simulink model "Lab6_2017B5A30983P_Midpoint_Fullwave"  (R2019b)
settings: Solver=ode15s  StartTime=0.0  StopTime=0.06  RelTol=1e-3
libraries: powerlib x8, powerlib_meascontrol x2
settings Model: Creator=swaga  LastModifiedBy=swaga

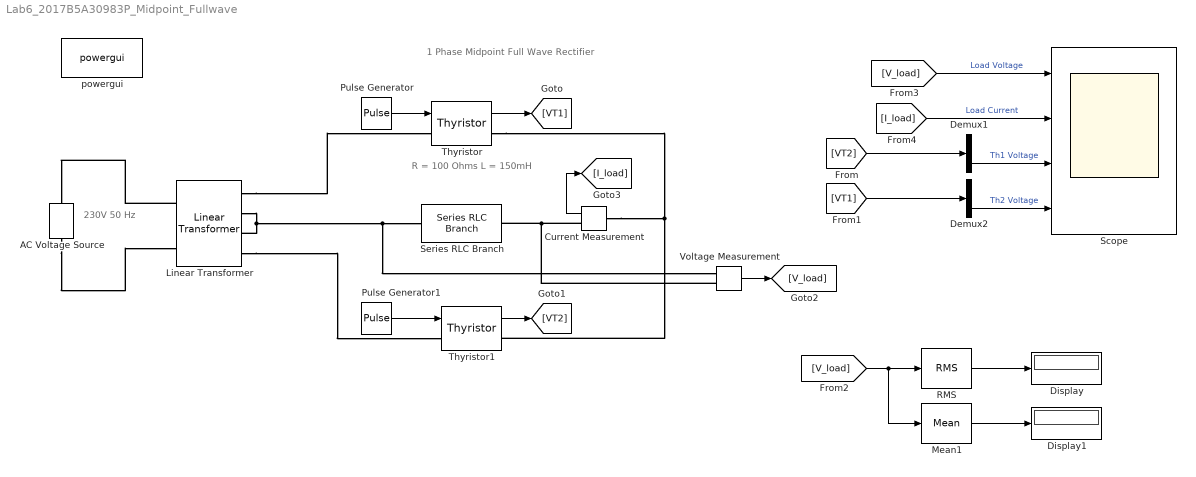
== system Lab6_2017B5A30983P_Midpoint_Fullwave ==
  note: R = 100 Ohms
      | L = 150mH
  note: 1 Phase Midpoint Full Wave Rectifier
  note: 230V
      | 50 Hz
  AC Voltage Source : powerlib/Electrical Sources/AC Voltage Source  Amplitude=230  Phase=0  Frequency=50  SampleTime=0  Measurements=None  BusType=swing  Pref=10e3  Qref=0  Qmin=-inf  Qmax=+inf
      settings: SourceProductName=Simscape Electrical
  Current Measurement : powerlib/Measurements/Current Measurement  PhasorSimulation=off  OutputType=Complex  PSBequivalent=0
      settings: SourceProductName=Simscape Electrical
  Demux1 : Demux  Outputs=2
  Demux2 : Demux  Outputs=2
  Display : Display
  Display1 : Display
  Linear Transformer : powerlib/Elements/Linear Transformer  UNITS=pu  NominalPower=[250e6 50]  winding1=[230 0.002 0.08]  winding2=[12 0.002 0]  ThreeWindings=on  winding3=[12 0.002 0]  RmLm=[ 500 500 ]  Measurements=None  DataType=off
      settings: SourceProductName=Simscape Electrical
  Mean1 : powerlib_meascontrol/Measurements/Mean  Freq=50  Vinit=0  Ts=0
      settings: SourceProductName=Simscape Electrical
  Pulse Generator : DiscretePulseGenerator  PulseType=Time based  Period=0.02  PulseWidth=5  PhaseDelay=2.5e-3
  Pulse Generator1 : DiscretePulseGenerator  PulseType=Time based  Period=0.02  PulseWidth=5  PhaseDelay=12.5e-3
  RMS : powerlib_meascontrol/Measurements/RMS  TrueRMS=on  Freq=50  RMSInit=120  Ts=0
      settings: SourceProductName=Simscape Electrical
  Scope : Scope  NumInputPorts=4
  Series RLC Branch : powerlib/Elements/Series RLC Branch  LConnTagsString=__new0  RConnTagsString=__new0  BranchType=R  Resistance=100  Inductance=150e-3  SetiL0=off  InitialCurrent=0  Capacitance=1e-6  Setx0=off  InitialVoltage=0  Measurements=None
      settings: SourceProductName=Simscape Electrical
  Thyristor : powerlib/Power Electronics/Thyristor  Ron=0.001  Lon=0  Vf=0.8  IC=0  Rs=500  Cs=250e-9  Measurements=on
      settings: SourceProductName=Simscape Electrical
  Thyristor1 : powerlib/Power Electronics/Thyristor  Ron=0.001  Lon=0  Vf=0.8  IC=0  Rs=500  Cs=250e-9  Measurements=on
      settings: SourceProductName=Simscape Electrical
  Voltage Measurement : powerlib/Measurements/Voltage Measurement  PhasorSimulation=off  OutputType=Complex  PSBequivalent=0
      settings: SourceProductName=Simscape Electrical
  powergui : powerlib/powergui  Priority=1  SimulationMode=Continuous  SampleTime=50e-6  frequency=60  Iterations=50  frequencyindice=50  Pbase=100e6  ErrMax=1e-4  UnitsV=kV  UnitsW=MW  buscounter=0  FunctionMessages=off  echomessages=off  EnableUseOfTLC=off  CurrentSourceSwitches=off  DisableSnubberDevices=off  DisableRonSwitches=off  DisableVfSwitches=off  DisplayEquations=off  AutomaticDiscreteSolvers=off  SolverType=Tustin/Backward Euler (TBE)  Interpol=off  ExternalGateDelay=off  methode=off  Ts=100  x0status=blocks  SPID=on  SwTol=0  HookPort=off  NonlinearTolerance=1e-4  nMaxIteration=100  ContinueOnMaxIteration=off  RestoreLinks=warning  ResistiveCurrentMeasurement=off  Frange=[0:2:500]  Ylog=off  Xlog=on  ShowGrid=off  save=off  variable=ZData  structure=0  ZoomFFT=off  StartTime=0.0  cycles=1  DisplayStyle=1  fundamental=60  FreqAxis=off  MaxFrequency=1000  frequencyindicesteady=1  RmsSteady=1  display=off
      settings: SourceProductName=Simscape Electrical
  wires:
  Pulse Generator/1 -> Thyristor/1
  Pulse Generator1/1 -> Thyristor1/1
  Thyristor/1 -> [VT1]
  Thyristor1/1 -> [VT2]
  Voltage Measurement/1 -> [V_load]
  Current Measurement/1 -> [I_load]
  Mean1/1 -> Display1/1
  [V_load] -> Mean1/1, RMS/1
  RMS/1 -> Display/1
  [VT1] -> Demux2/1
  [VT2] -> Demux1/1
  [I_load] -> Scope/2  "Load Current"
  [V_load] -> Scope/1  "Load Voltage"
  Demux2/2 -> Scope/4  "Th2 Voltage"
  Demux1/2 -> Scope/3  "Th1 Voltage"
  connections:
  Thyristor/RConn1 -- Current Measurement/LConn1 -- Thyristor1/RConn1
  Current Measurement/RConn1 -- Series RLC Branch/RConn1 -- Voltage Measurement/LConn1
  Linear Transformer/RConn2 -- Linear Transformer/RConn3 -- Voltage Measurement/LConn2 -- Series RLC Branch/LConn1
  Linear Transformer/RConn4 -- Thyristor1/LConn1
  Linear Transformer/RConn1 -- Thyristor/LConn1
  Linear Transformer/LConn1 -- AC Voltage Source/RConn1
  AC Voltage Source/LConn1 -- Linear Transformer/LConn2
